simulink model "simulink_final"  (R2021a)
settings: Solver=FixedStepAuto  StartTime=0.0  StopTime=10.0  FixedStep=1e-3  RelTol=1e-3  EnableMultiTasking=on
undefined symbols (not defined in the file): a, A0, A1, b, c, D0, D1, D10, D11, D12, D13, D2, D3, D4, D5, D6, D7, D8, D9, magnitude, PTA0, PTA1, PTA2, PTB2, PTB23, PTB3, PTB9, PTC16, PTC17, PTC2, PTC3, PTC4, PTD0, PTD1, PTD2, PTD3
libraries: frdmk64flib x34, dspstat3 x2, hdlsllib x2, etargetslib x2, simulink x1
settings Model: ExtModeTrigDuration=5  Creator=14610  LastModifiedBy=微星
settings SolverCC: AlgebraicLoopSolver=TrustRegion
settings OptimizationCC: EnhancedBackFolding=on  PassReuseOutputArgsAs=Individual arguments  ZeroExternalMemoryAtStartup=off  ZeroInternalMemoryAtStartup=off  MaxStackSize=64  OptimizeBlockOrder=speed  DifferentSizesBufferReuse=on  OptimizationCustomize=off  EfficientTunableParamExpr=on
settings DebuggingCC: ParameterTunabilityLossMsg=error  SFMachineParentedDataDiag=warning
settings HardwareCC: ProdBitPerPointer=32  ProdBitPerSizeT=32  ProdBitPerPtrDiffT=32  ProdLargestAtomicInteger=Long  ProdLargestAtomicFloat=Double  ProdWordSize=32  ProdHWDeviceType=ARM Compatible->ARM Cortex  UseEmbeddedCoderFeatures=off
settings SFSimCC: MATLABDynamicMemAlloc=off
settings RTWCC: SystemTargetFile=ert.tlc  HardwareBoard=NXP FRDM-K64F  TLCOptions="-aInlineSetEventsForThisBaseRateFcn=TLC_FALSE -aSuppressMultiTaskScheduler=TLC_FALSE  -aRateBasedStepFcn=0"  TemplateMakefile=ert_default_tmf  Toolchain=GNU Tools for ARM Embedded Processors
settings CodeAppCC: ForceParamTrailComments=on  IgnoreCustomStorageClasses=off  OperatorAnnotations=on  SimulinkDataObjDesc=on  SFDataObjDesc=on  InsertBlockDesc=on
settings ERTTargetCC: SupportNonInlinedSFcns=on

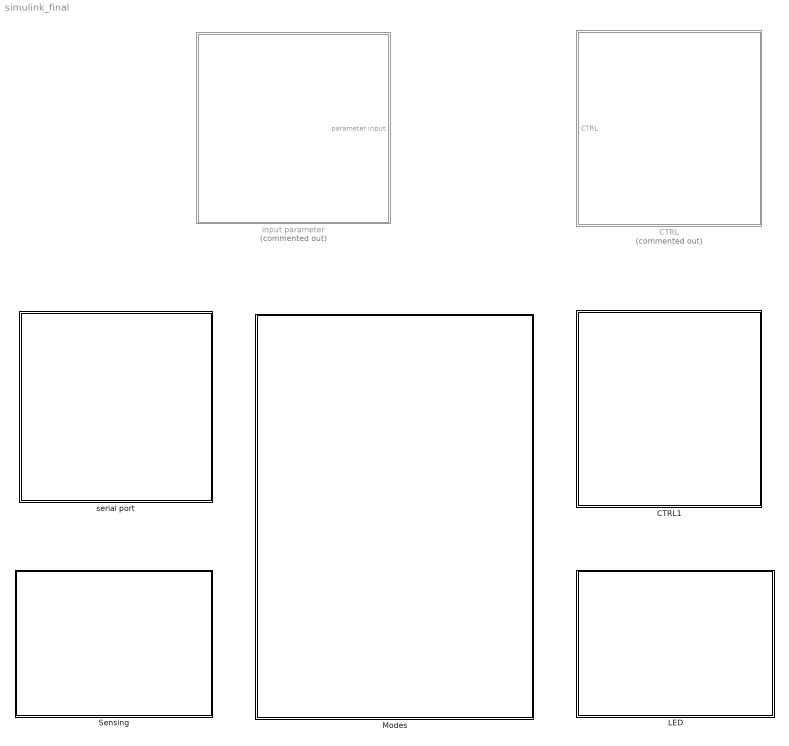
== system simulink_final ==
  CTRL : Subsystem  Commented=on
  CTRL1 : Subsystem
  LED : Subsystem
  Modes : Subsystem
  Sensing : Subsystem
  input parameter : Subsystem  Commented=on
  serial port : Subsystem

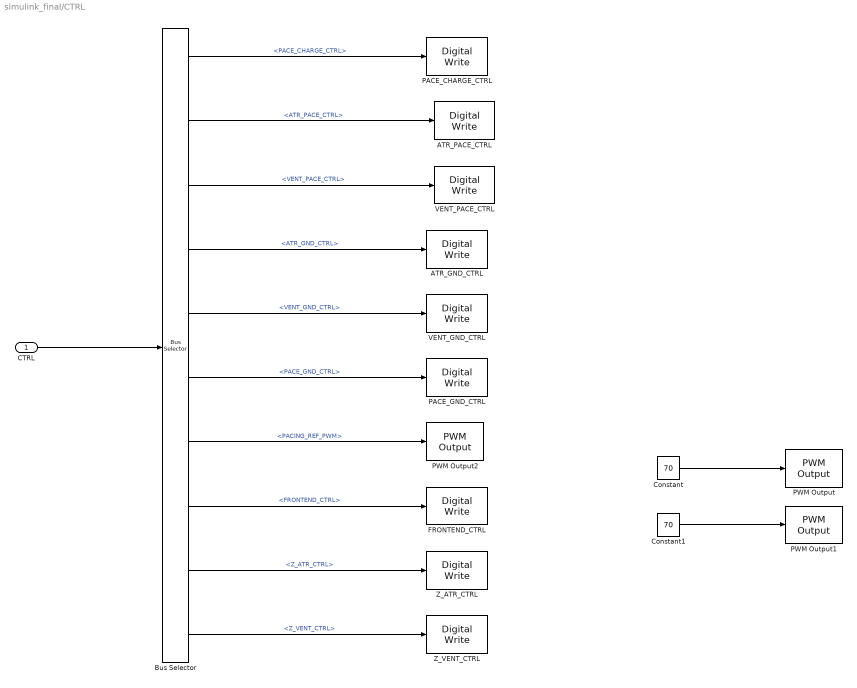
== system simulink_final/CTRL ==
  CTRL : Inport
  ATR_GND_CTRL : frdmk64flib/Digital Write  Whichpin=PTD2 (D11)
  ATR_PACE_CTRL : frdmk64flib/Digital Write  Whichpin=PTA0 (D8)
  Bus Selector : BusSelector  OutputSignals=PACE_CHARGE_CTRL,ATR_PACE_CTRL,VENT_PACE_CTRL,ATR_GND_CTRL,VENT_GND_CTRL,PACE_GND_CTRL,PACING_REF_PWM,FRONTEND_CTRL,Z_ATR_CTRL,Z_VENT_CTRL
  Constant : Constant  Value=70
  Constant1 : Constant  Value=70
  FRONTEND_CTRL : frdmk64flib/Digital Write  Whichpin=PTD1 (D13)
  PACE_CHARGE_CTRL : frdmk64flib/Digital Write  Whichpin=PTB9 (D2)
  PACE_GND_CTRL : frdmk64flib/Digital Write  Whichpin=PTD0 (D10)
  PWM Output : frdmk64flib/PWM Output  Whichpin=PTC2 (D6)  InitialFrequency=2000  InitialDutyCycle=30
  PWM Output1 : frdmk64flib/PWM Output  Whichpin=PTA1 (D3)  InitialFrequency=2000  InitialDutyCycle=30
  PWM Output2 : frdmk64flib/PWM Output  Whichpin=PTA2 (D5)  InitialFrequency=2000  InitialDutyCycle=30
  VENT_GND_CTRL : frdmk64flib/Digital Write  Whichpin=PTD3 (D12)
  VENT_PACE_CTRL : frdmk64flib/Digital Write  Whichpin=PTC4 (D9)
  Z_ATR_CTRL : frdmk64flib/Digital Write  Whichpin=PTB23 (D4)
  Z_VENT_CTRL : frdmk64flib/Digital Write  Whichpin=PTC3 (D7)
  wires:
  CTRL/1 -> Bus Selector/1
  Bus Selector/2 -> ATR_PACE_CTRL/1  "<ATR_PACE_CTRL>"
  Bus Selector/1 -> PACE_CHARGE_CTRL/1  "<PACE_CHARGE_CTRL>"
  Bus Selector/3 -> VENT_PACE_CTRL/1  "<VENT_PACE_CTRL>"
  Bus Selector/4 -> ATR_GND_CTRL/1  "<ATR_GND_CTRL>"
  Bus Selector/5 -> VENT_GND_CTRL/1  "<VENT_GND_CTRL>"
  Bus Selector/6 -> PACE_GND_CTRL/1  "<PACE_GND_CTRL>"
  Bus Selector/7 -> PWM Output2/1  "<PACING_REF_PWM>"
  Bus Selector/8 -> FRONTEND_CTRL/1  "<FRONTEND_CTRL>"
  Bus Selector/9 -> Z_ATR_CTRL/1  "<Z_ATR_CTRL>"
  Bus Selector/10 -> Z_VENT_CTRL/1  "<Z_VENT_CTRL>"
  Constant/1 -> PWM Output/1
  Constant1/1 -> PWM Output1/1

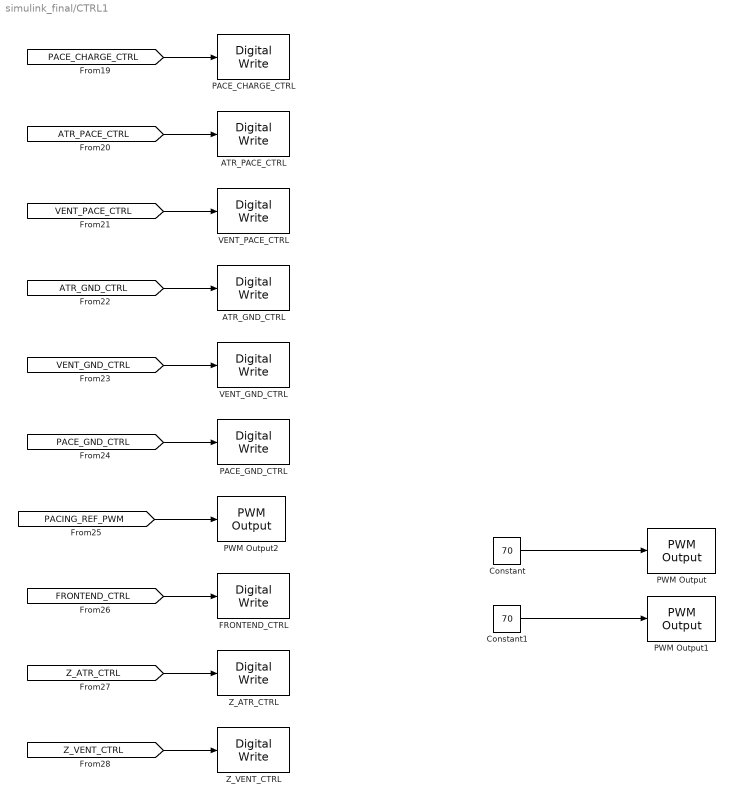
== system simulink_final/CTRL1 ==
  ATR_GND_CTRL : frdmk64flib/Digital Write  Whichpin=PTD2 (D11)
  ATR_PACE_CTRL : frdmk64flib/Digital Write  Whichpin=PTA0 (D8)
  Constant : Constant  Value=70
  Constant1 : Constant  Value=70
  FRONTEND_CTRL : frdmk64flib/Digital Write  Whichpin=PTD1 (D13)
  PACE_CHARGE_CTRL : frdmk64flib/Digital Write  Whichpin=PTB9 (D2)
  PACE_GND_CTRL : frdmk64flib/Digital Write  Whichpin=PTD0 (D10)
  PWM Output : frdmk64flib/PWM Output  Whichpin=PTC2 (D6)  InitialFrequency=2000  InitialDutyCycle=30
  PWM Output1 : frdmk64flib/PWM Output  Whichpin=PTA1 (D3)  InitialFrequency=2000  InitialDutyCycle=30
  PWM Output2 : frdmk64flib/PWM Output  Whichpin=PTA2 (D5)  InitialFrequency=2000  InitialDutyCycle=30
  VENT_GND_CTRL : frdmk64flib/Digital Write  Whichpin=PTD3 (D12)
  VENT_PACE_CTRL : frdmk64flib/Digital Write  Whichpin=PTC4 (D9)
  Z_ATR_CTRL : frdmk64flib/Digital Write  Whichpin=PTB23 (D4)
  Z_VENT_CTRL : frdmk64flib/Digital Write  Whichpin=PTC3 (D7)
  wires:
  Constant/1 -> PWM Output/1
  Constant1/1 -> PWM Output1/1
  [PACE_CHARGE_CTRL] -> PACE_CHARGE_CTRL/1
  [ATR_PACE_CTRL] -> ATR_PACE_CTRL/1
  [VENT_PACE_CTRL] -> VENT_PACE_CTRL/1
  [ATR_GND_CTRL] -> ATR_GND_CTRL/1
  [VENT_GND_CTRL] -> VENT_GND_CTRL/1
  [PACE_GND_CTRL] -> PACE_GND_CTRL/1
  [Z_VENT_CTRL] -> Z_VENT_CTRL/1
  [FRONTEND_CTRL] -> FRONTEND_CTRL/1
  [Z_ATR_CTRL] -> Z_ATR_CTRL/1
  [PACING_REF_PWM] -> PWM Output2/1

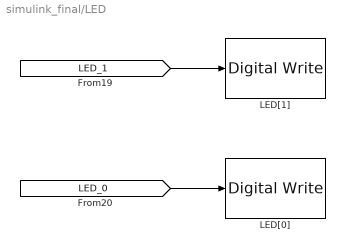
== system simulink_final/LED ==
  LED[0] : frdmk64flib/Digital Write  Whichpin=RED_LED
  LED[1] : frdmk64flib/Digital Write  Whichpin=GREEN_LED
  wires:
  [LED_1] -> LED[1]/1
  [LED_0] -> LED[0]/1

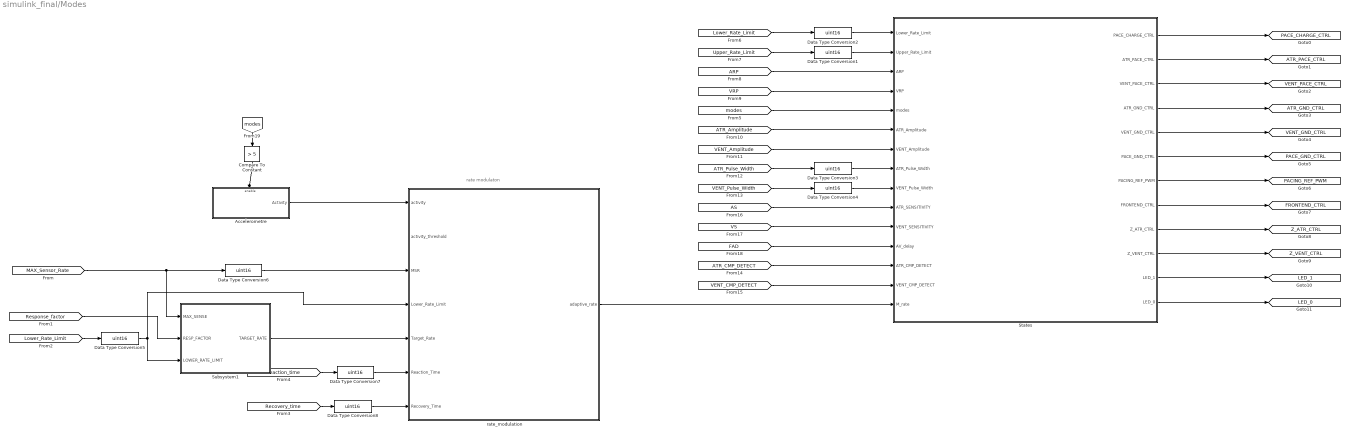
== system simulink_final/Modes ==
  note: rate modulaton
  Accelerometre : Subsystem
  Compare To Constant : simulink/Logic and Bit Operations/Compare To Constant  relop=>  const=5  OutDataTypeStr=boolean
  Data Type Conversion{1..8} (8 alike) : DataTypeConversion  OutDataTypeStr=uint16
  States : Stateflow chart
      settings: PortSchema="{\"entries\":[{\"content\":{\"sides\":[{\"content\":{\"connectorIds\":[\"In1\",\"In2\",\"In3\",\"In4\",\"In5\",\"In8\",\"In9\",\"In10\",\"In11\",\"In13\",\"In14\",\"In12\",\"In6\",\"In7\",\"In15\"]},\"type\":\"ConnectorPlacement.EquallySpacedRectSide\",\"uuid\":\"1bf89235-5b2a-4a6d-8fd1-80cb7ace4fe1\"},{\"content\":{\"connectorIds\":[\"Out1\",\"Out2\",\"Out3\",\"Out4\",\"Out5\",\"Out6\",\"Out7\",\"Out8\",\"Out9\",\"Out10\",\"Out11\",\"Out12\"],\"side\":\"RIGHT\"},\"type\":\"ConnectorPlacement.EquallySpacedRectSide\",\"uuid\":\"14ca63ff-77f8-4fed-b6c6-f39543f8346a\"},{\"content\":{\"connectorIds\":[],\"side\":\"TOP\"},\"type\":\"ConnectorPlacement.EquallySpacedRectSide\",\"uuid\":\"86655f59-e294-4cfd-9413-44776565e2db\"}]},\"type\":\"ConnectorPlacement.EquallySpacedConnector\",\"uuid\":\"c44c9a5a-010f-4149-9f0b-fe431661db61\"}],\"packageUris\":[\"http://schema.mathworks.com/mf0/Connector/R2020b\"],\"version\":\"1.0\"}"
  Subsystem1 : Subsystem
  rate_modulation : Stateflow chart  TreatAsAtomicUnit=on
  tag scope: ATR_GND_CTRL=global, ATR_PACE_CTRL=global, FRONTEND_CTRL=global, LED_0=global, LED_1=global, PACE_CHARGE_CTRL=global, PACE_GND_CTRL=global, PACING_REF_PWM=global, VENT_GND_CTRL=global, VENT_PACE_CTRL=global, Z_ATR_CTRL=global, Z_VENT_CTRL=global
  wires:
  [modes] -> States/5(modes)
  [VRP] -> States/4(VRP)
  [ARP] -> States/3(ARP)
  [VENT_Pulse_Width] -> Data Type Conversion4/1
  [VENT_Amplitude] -> States/9(VENT_Amplitude)
  [ATR_Amplitude] -> States/8(ATR_Amplitude)
  [Upper_Rate_Limit] -> Data Type Conversion1/1
  [Lower_Rate_Limit] -> Data Type Conversion2/1
  States/1(PACE_CHARGE_CTRL) -> [PACE_CHARGE_CTRL]
  States/2(ATR_PACE_CTRL) -> [ATR_PACE_CTRL]
  States/3(VENT_PACE_CTRL) -> [VENT_PACE_CTRL]
  States/4(ATR_GND_CTRL) -> [ATR_GND_CTRL]
  States/5(VENT_GND_CTRL) -> [VENT_GND_CTRL]
  States/6(PACE_GND_CTRL) -> [PACE_GND_CTRL]
  States/7(PACING_REF_PWM) -> [PACING_REF_PWM]
  States/8(FRONTEND_CTRL) -> [FRONTEND_CTRL]
  States/9(Z_ATR_CTRL) -> [Z_ATR_CTRL]
  States/10(Z_VENT_CTRL) -> [Z_VENT_CTRL]
  [ATR_Pulse_Width] -> Data Type Conversion3/1
  [AS] -> States/13(ATR_SENSITIVITY)
  [VS] -> States/14(VENT_SENSITIVITY)
  [FAD] -> States/12(AV_delay)
  [MAX_Sensor_Rate] -> Subsystem1/1(MAX_SENSE), Data Type Conversion6/1
  [Response_factor] -> Subsystem1/2(RESP_FACTOR)
  [Lower_Rate_Limit] -> Data Type Conversion5/1
  [ATR_CMP_DETECT] -> States/6(ATR_CMP_DETECT)
  [VENT_CMP_DETECT] -> States/7(VENT_CMP_DETECT)
  States/11(LED_1) -> [LED_1]
  States/12(LED_0) -> [LED_0]
  [modes] -> Compare To Constant/1
  Compare To Constant/1 -> Accelerometre/Enable
  Data Type Conversion2/1 -> States/1(Lower_Rate_Limit)
  Data Type Conversion1/1 -> States/2(Upper_Rate_Limit)
  Data Type Conversion3/1 -> States/10(ATR_Pulse_Width)
  Data Type Conversion4/1 -> States/11(VENT_Pulse_Width)
  Data Type Conversion5/1 -> Subsystem1/3(LOWER_RATE_LIMIT), rate_modulation/4(Lower_Rate_Limit)
  Accelerometre/1(Activity) -> rate_modulation/1(activity)
  Subsystem1/1(TARGET_RATE) -> rate_modulation/5(Target_Rate)
  [Reaction_time] -> Data Type Conversion7/1
  [Recovery_time] -> Data Type Conversion8/1
  Data Type Conversion6/1 -> rate_modulation/3(MSR)
  Data Type Conversion7/1 -> rate_modulation/6(Reaction_Time)
  Data Type Conversion8/1 -> rate_modulation/7(Recovery_Time)
  rate_modulation/1(adaptive_rate) -> States/15(M_rate)

== system simulink_final/Sensing ==
  ATR_CMP_ DETECT : frdmk64flib/Digital Read  Whichpin=PTC16 (D0)  SampleTime=-1
  VENT_CMP_DETECT : frdmk64flib/Digital Read  Whichpin=PTC17 (D1)  SampleTime=-1
  tag scope: ATR_CMP_DETECT=global, VENT_CMP_DETECT=global
  wires:
  ATR_CMP_ DETECT/1 -> [ATR_CMP_DETECT]  "ATR_CMP_ DETECT"
  VENT_CMP_DETECT/1 -> [VENT_CMP_DETECT]  "VENT_CMP_ DETECT"

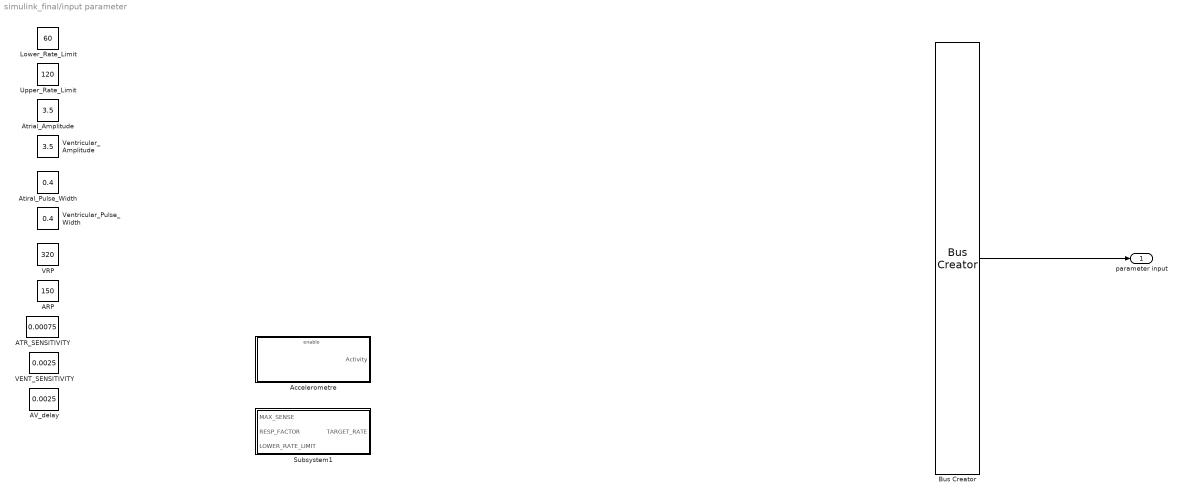
== system simulink_final/input parameter ==
  ARP : Constant  Value=150
  ATR_SENSITIVITY : Constant  Value=0.00075
  AV_delay : Constant  Value=0.0025
  Accelerometre : Subsystem
  Atiral_Pulse_Width : Constant  Value=0.4
  Atrial_Amplitude : Constant  Value=3.5
  Bus Creator : BusCreator  Inputs=12
  Lower_Rate_Limit : Constant  Value=60
  Subsystem1 : Subsystem
  Upper_Rate_Limit : Constant  Value=120
  VENT_SENSITIVITY : Constant  Value=0.0025
  VRP : Constant  Value=320
  Ventricular_Amplitude : Constant  Value=3.5
  Ventricular_Pulse_Width : Constant  Value=0.4
  parameter input : Outport
  wires:
  Bus Creator/1 -> parameter input/1
  ? -> Bus Creator/1  "modes"
  ? -> Bus Creator/2
  ? -> Bus Creator/3
  ? -> Bus Creator/4
  ? -> Bus Creator/5
  ? -> Bus Creator/6
  ? -> Bus Creator/7
  ? -> Bus Creator/8
  ? -> Bus Creator/9

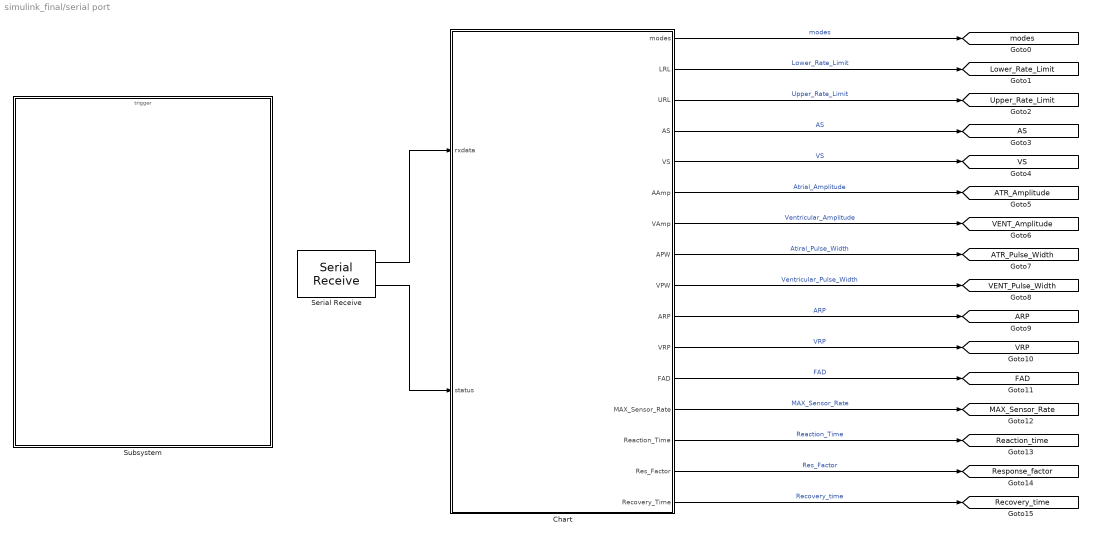
== system simulink_final/serial port ==
  Chart : Stateflow chart  TreatAsAtomicUnit=on
      settings: PortSchema="{\"entries\":[{\"content\":{\"sides\":[{\"content\":{\"connectorIds\":[\"In1\",\"In2\"]},\"type\":\"ConnectorPlacement.EquallySpacedRectSide\",\"uuid\":\"355b2c62-f4ab-4f69-b4c3-58c4813cdbb8\"},{\"content\":{\"connectorIds\":[\"Out1\",\"Out2\",\"Out14\",\"Out15\",\"Out16\",\"Out3\",\"Out4\",\"Out5\",\"Out6\",\"Out7\",\"Out8\",\"Out9\",\"Out10\",\"Out11\",\"Out12\",\"Out13\"],\"side\":\"RIGHT\"},\"type\":\"ConnectorPlacement.EquallySpacedRectSide\",\"uuid\":\"e39f9fe7-8151-4d9f-b318-f4c2a6150d39\"},{\"content\":{\"connectorIds\":[],\"side\":\"TOP\"},\"type\":\"ConnectorPlacement.EquallySpacedRectSide\",\"uuid\":\"4076b67e-1825-4591-a111-6e489612a839\"}]},\"type\":\"ConnectorPlacement.EquallySpacedConnector\",\"uuid\":\"92306b88-4ce7-4751-b58c-bc5096b575c6\"}],\"packageUris\":[\"http://schema.mathworks.com/mf0/Connector/R2020b\"],\"version\":\"1.0\"}"
  Serial Receive : frdmk64flib/Serial Receive  SCIModule=0  Baudrate=uint32(9600)  Parity=None  StopBits=1  HardwareFlowControl=None  ByteOrder=LittleEndian  DataType=uint8  DataLength=21  BlockingMode=off  OutputStatus=on  SampleTime=-1
  Subsystem : Subsystem
  tag scope: ARP=global, AS=global, ATR_Amplitude=global, ATR_Pulse_Width=global, FAD=global, Lower_Rate_Limit=global, MAX_Sensor_Rate=global, Reaction_time=global, Recovery_time=global, Response_factor=global, Upper_Rate_Limit=global, VENT_Amplitude=global, VENT_Pulse_Width=global, VRP=global, VS=global, modes=global
  wires:
  Chart/1(modes) -> [modes]  "modes"
  Chart/2(LRL) -> [Lower_Rate_Limit]  "Lower_Rate_Limit"
  Chart/14(URL) -> [Upper_Rate_Limit]  "Upper_Rate_Limit"
  Chart/15(AS) -> [AS]  "AS"
  Chart/16(VS) -> [VS]  "VS"
  Chart/3(AAmp) -> [ATR_Amplitude]  "Atrial_Amplitude"
  Chart/4(VAmp) -> [VENT_Amplitude]  "Ventricular_Amplitude"
  Chart/5(APW) -> [ATR_Pulse_Width]  "Atiral_Pulse_Width"
  Chart/6(VPW) -> [VENT_Pulse_Width]  "Ventricular_Pulse_Width"
  Chart/7(ARP) -> [ARP]  "ARP"
  Chart/8(VRP) -> [VRP]  "VRP"
  Chart/9(FAD) -> [FAD]  "FAD"
  Chart/10(MAX_Sensor_Rate) -> [MAX_Sensor_Rate]  "MAX_Sensor_Rate"
  Chart/11(Reaction_Time) -> [Reaction_time]  "Reaction_Time"
  Chart/12(Res_Factor) -> [Response_factor]  "Res_Factor"
  Chart/13(Recovery_Time) -> [Recovery_time]  "Recovery_time"
  Serial Receive/1 -> Chart/1(rxdata)
  Serial Receive/2 -> Chart/2(status)

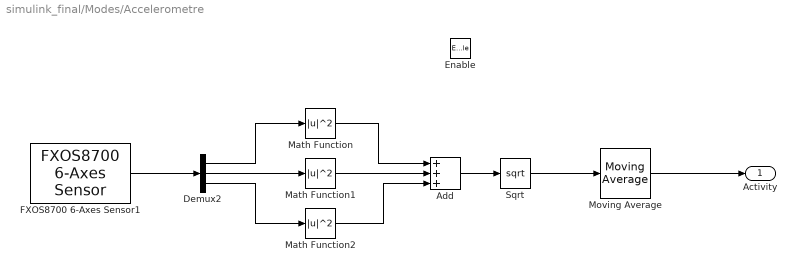
== system simulink_final/Modes/Accelerometre ==
  Enable : EnablePort
  Add : Sum  Inputs=+++
  Demux2 : Demux  Outputs=3
  FXOS8700 6-Axes Sensor1 : frdmk64flib/FXOS8700 6-Axes Sensor  Activesensor=Accelerometer only  ODR=100Hz  HybridODR=400Hz  Accelfullrange=-4g to +4g  SampleTime=1/100
  Math Function : Math  Operator=magnitude^2  SignedPower=on  OutDataTypeStr=double  SaturateOnIntegerOverflow=on
  Math Function1 : Math  Operator=magnitude^2  SignedPower=on  OutDataTypeStr=double  SaturateOnIntegerOverflow=on
  Math Function2 : Math  Operator=magnitude^2  SignedPower=on  OutDataTypeStr=double  SaturateOnIntegerOverflow=on
  Moving Average : dspstat3/Moving Average  Method=Sliding window  ForgettingFactorPort=off  SpecifyWindowLength=on  WindowLength=4  ForgettingFactor=0.9  SimulateUsing=Code generation
  Sqrt : Sqrt  SaturateOnIntegerOverflow=on
  Activity : Outport  OutDataTypeStr=double  SourceOfInitialOutputValue=Input signal
  wires:
  Sqrt/1 -> Moving Average/1
  FXOS8700 6-Axes Sensor1/1 -> Demux2/1
  Math Function/1 -> Add/1
  Add/1 -> Sqrt/1
  Math Function2/1 -> Add/3
  Demux2/2 -> Math Function1/1
  Math Function1/1 -> Add/2
  Demux2/1 -> Math Function/1
  Demux2/3 -> Math Function2/1
  Moving Average/1 -> Activity/1

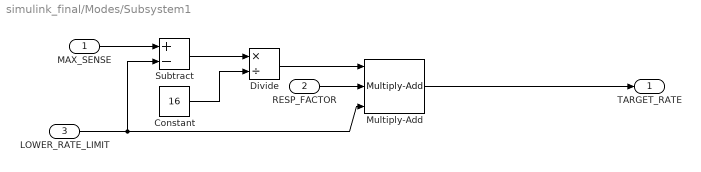
== system simulink_final/Modes/Subsystem1 ==
  MAX_SENSE : Inport
  RESP_FACTOR : Inport  Port=2
  LOWER_RATE_LIMIT : Inport  Port=3
  Constant : Constant  Value=16
  Divide : Product  Inputs=*/
  Multiply-Add : hdlsllib/HDL Operations/Multiply-Add  Function=c+(a.*b)  datatype=uint16  RndMeth=Nearest  DoSatur=off  FMA=off
      settings: SourceProductBaseCode=SL
  Subtract : Sum  Inputs=+-
  TARGET_RATE : Outport  OutDataTypeStr=uint16  SourceOfInitialOutputValue=Input signal
  wires:
  MAX_SENSE/1 -> Subtract/1
  Subtract/1 -> Divide/1
  Constant/1 -> Divide/2
  Divide/1 -> Multiply-Add/1
  RESP_FACTOR/1 -> Multiply-Add/2
  Multiply-Add/1 -> TARGET_RATE/1
  LOWER_RATE_LIMIT/1 -> Subtract/2, Multiply-Add/3

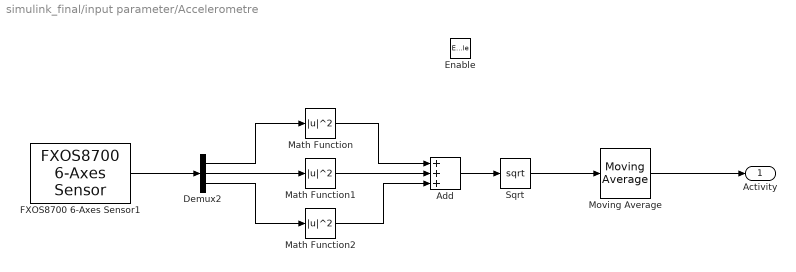
== system simulink_final/input parameter/Accelerometre ==
  Enable : EnablePort
  Add : Sum  Inputs=+++
  Demux2 : Demux  Outputs=3
  FXOS8700 6-Axes Sensor1 : frdmk64flib/FXOS8700 6-Axes Sensor  Activesensor=Accelerometer only  ODR=100Hz  HybridODR=400Hz  Accelfullrange=-4g to +4g  SampleTime=1/100
  Math Function : Math  Operator=magnitude^2  SignedPower=on  OutDataTypeStr=double  SaturateOnIntegerOverflow=on
  Math Function1 : Math  Operator=magnitude^2  SignedPower=on  OutDataTypeStr=double  SaturateOnIntegerOverflow=on
  Math Function2 : Math  Operator=magnitude^2  SignedPower=on  OutDataTypeStr=double  SaturateOnIntegerOverflow=on
  Moving Average : dspstat3/Moving Average  Method=Sliding window  ForgettingFactorPort=off  SpecifyWindowLength=on  WindowLength=4  ForgettingFactor=0.9  SimulateUsing=Code generation
  Sqrt : Sqrt  SaturateOnIntegerOverflow=on
  Activity : Outport  OutDataTypeStr=double  SourceOfInitialOutputValue=Input signal
  wires:
  Sqrt/1 -> Moving Average/1
  FXOS8700 6-Axes Sensor1/1 -> Demux2/1
  Math Function/1 -> Add/1
  Add/1 -> Sqrt/1
  Math Function2/1 -> Add/3
  Demux2/2 -> Math Function1/1
  Math Function1/1 -> Add/2
  Demux2/1 -> Math Function/1
  Demux2/3 -> Math Function2/1
  Moving Average/1 -> Activity/1

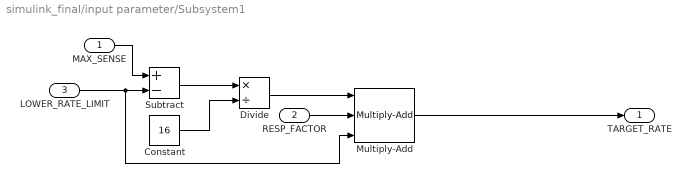
== system simulink_final/input parameter/Subsystem1 ==
  MAX_SENSE : Inport
  RESP_FACTOR : Inport  Port=2
  LOWER_RATE_LIMIT : Inport  Port=3
  Constant : Constant  Value=16
  Divide : Product  Inputs=*/
  Multiply-Add : hdlsllib/HDL Operations/Multiply-Add  Function=c+(a.*b)  datatype=uint16  RndMeth=Nearest  DoSatur=off  FMA=off
      settings: SourceProductBaseCode=SL
  Subtract : Sum  Inputs=+-
  TARGET_RATE : Outport  OutDataTypeStr=uint16  SourceOfInitialOutputValue=Input signal
  wires:
  MAX_SENSE/1 -> Subtract/1
  LOWER_RATE_LIMIT/1 -> Multiply-Add/3, Subtract/2
  Subtract/1 -> Divide/1
  Constant/1 -> Divide/2
  Divide/1 -> Multiply-Add/1
  RESP_FACTOR/1 -> Multiply-Add/2
  Multiply-Add/1 -> TARGET_RATE/1

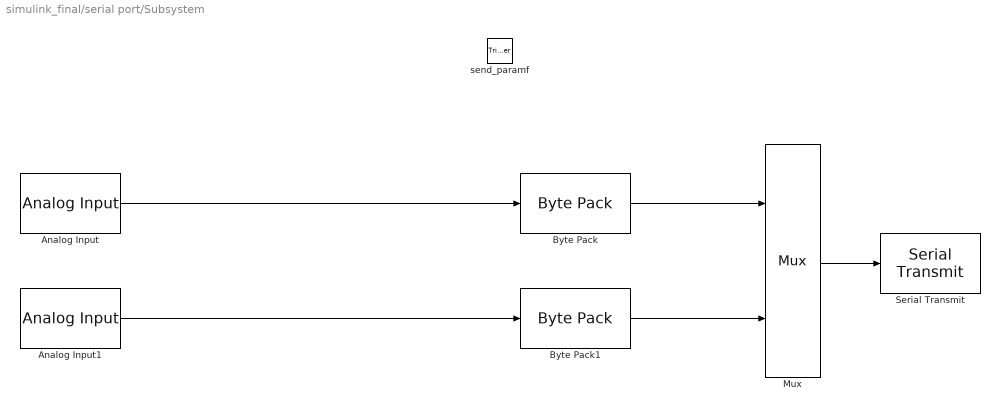
== system simulink_final/serial port/Subsystem ==
  send_paramf : TriggerPort  TriggerType=function-call  IsSimulinkFunction=on  FunctionName=send_paramf  VariantControl=(inherit)  PortDimensions=1
  Analog Input : frdmk64flib/Analog Input  Whichpin=PTB2 (A0)  SampleTime=-1
  Analog Input1 : frdmk64flib/Analog Input  Whichpin=PTB3 (A1)  SampleTime=-1
  Byte Pack : etargetslib/Byte Pack  datatypes={'double'}  byteAlign=1
  Byte Pack1 : etargetslib/Byte Pack  datatypes={'double'}  byteAlign=1
  Mux : Mux  Inputs=2
  Serial Transmit : frdmk64flib/Serial Transmit  SCIModule=0  Baudrate=uint32(9600)  Parity=None  StopBits=1  HardwareFlowControl=None  ByteOrder=LittleEndian  BlockingMode=on  OutputStatus=off
  wires:
  Byte Pack/1 -> Mux/1
  Byte Pack1/1 -> Mux/2
  Mux/1 -> Serial Transmit/1
  Analog Input/1 -> Byte Pack/1
  Analog Input1/1 -> Byte Pack1/1

== stateflow chart simulink_final/Modes/States ==
  note: will leave the defult state if recieve any changes in parameter mode
  state Defult
    entry:
    PACE_CHARGE_CTRL=0;
    PACE_GND_CTRL = 0;
    ATR_PACE_CTRL = 0;
    ATR_GND_CTRL = 0;
    VENT_PACE_CTRL = 0;
    VENT_GND_CTRL = 0;
    LED_1 = 1;
    %ATR_CMP_REF_PWM = ATR_SENSITIVITY*100/3.3;
    %VENT_CMP_REF_PWM = VENT_SENSITIVITY*100/3.3;
  note: will go back to defult sate if the any new changes in parameter mode
  state AAIR
    state AAIR
      entry:
      PACE_CHARGE_CTRL=1;
      PACE_GND_CTRL = 1;
      ATR_PACE_CTRL = 0;
      ATR_GND_CTRL = 1;
      VENT_PACE_CTRL = 0;
      VENT_GND_CTRL = 0;
      PACING_REF_PWM = ATR_Amplitude;
      FRONTEND_CTRL = 1;
      Z_ATR_CTRL = 0;
      Z_VENT_CTRL = 0;
      LED_0 = 0;
      LED_1 = 0;
    note: charging C22 for the atrium pacing
    state Refractory_ATR
      entry:
      PACE_CHARGE_CTRL=1;
      PACE_GND_CTRL = 1;
      ATR_PACE_CTRL = 0;
      ATR_GND_CTRL = 1;
      VENT_PACE_CTRL = 0;
      VENT_GND_CTRL = 0;
      PACING_REF_PWM = ATR_Amplitude;
      FRONTEND_CTRL = 1;
      Z_ATR_CTRL = 0;
      Z_VENT_CTRL = 0;
      LED_0 = 0;
    state AAIR_PACING
      entry:
      PACE_CHARGE_CTRL=0;
      PACE_GND_CTRL = 1;
      ATR_PACE_CTRL = 1;
      ATR_GND_CTRL = 0;
      Z_ATR_CTRL = 0;
      Z_VENT_CTRL = 0;
      VENT_PACE_CTRL = 0;
      VENT_GND_CTRL = 0;
      LED_0 = 1;
    AAIR_PACING -> AAIR.AAIR : after(ATR_Pulse_Width,msec)
    AAIR.Refractory_ATR -> AAIR.AAIR [order 2] : [ATR_CMP_DETECT==1]
    AAIR.AAIR -> AAIR.Refractory_ATR [order 1] : after(ARP,msec)
    AAIR.Refractory_ATR -> AAIR_PACING [order 1] : after(60/M_rate * 1000 - ARP - ATR_Pulse_Width,msec)
  state VVIR
    state VVIR
      entry:
      PACE_CHARGE_CTRL=1;
      PACE_GND_CTRL = 1;
      ATR_PACE_CTRL = 0;
      ATR_GND_CTRL = 0;
      VENT_PACE_CTRL = 0;
      VENT_GND_CTRL = 1;
      PACING_REF_PWM = VENT_Amplitude;
      FRONTEND_CTRL = 1;
      Z_ATR_CTRL = 0;
      Z_VENT_CTRL = 0;
      LED_0 = 0;
      LED_1 = 0;
    note: charging C22 for the ventricle pacing
    state Refractory_VENT
      entry:
      PACE_CHARGE_CTRL=1;
      PACE_GND_CTRL = 1;
      ATR_PACE_CTRL = 0;
      ATR_GND_CTRL = 0;
      VENT_PACE_CTRL = 0;
      VENT_GND_CTRL = 1;
      PACING_REF_PWM = VENT_Amplitude;
      FRONTEND_CTRL = 1;
      Z_ATR_CTRL = 0;
      Z_VENT_CTRL = 0;
      LED_0 = 0;
    state VVIR_PACING
      entry:
      PACE_CHARGE_CTRL=0;
      PACE_GND_CTRL = 1;
      ATR_PACE_CTRL = 0;
      ATR_GND_CTRL = 0;
      Z_ATR_CTRL = 0;
      Z_VENT_CTRL = 0;
      VENT_PACE_CTRL = 1;
      VENT_GND_CTRL = 0;
      LED_0 = 1;
    VVIR.Refractory_VENT -> VVIR.VVIR [order 1] : [VENT_CMP_DETECT==1]
    VVIR_PACING -> VVIR.VVIR : after(VENT_Pulse_Width,msec)
    VVIR.VVIR -> VVIR.Refractory_VENT [order 2] : after(VRP,msec)
    VVIR.Refractory_VENT -> VVIR_PACING [order 2] : after(60/M_rate * 1000 - VRP - VENT_Pulse_Width,msec)
  state AOO
    state AOO
      entry:
      ATR_PACE_CTRL = 0;
      VENT_PACE_CTRL = 0;
      PACING_REF_PWM = ATR_Amplitude;
      PACE_CHARGE_CTRL = 1;
      PACE_GND_CTRL = 1;
      Z_ATR_CTRL = 0;
      Z_VENT_CTRL = 0;
      ATR_GND_CTRL = 1;
      VENT_GND_CTRL = 0;
      FRONTEND_CTRL = 0;
      LED_0 = 0;
      LED_1 = 0;
    note: charging C22 for the atrium pacing
    state AOO_PACING
      entry:
      PACE_CHARGE_CTRL=0;
      PACE_GND_CTRL = 1;
      ATR_PACE_CTRL = 1;
      ATR_GND_CTRL = 0;
      Z_ATR_CTRL = 0;
      Z_VENT_CTRL = 0;
      VENT_PACE_CTRL = 0;
      VENT_GND_CTRL = 0;
      LED_0 = 1;
    AOO.AOO -> AOO_PACING [order 2] : after(60000/Lower_Rate_Limit-ATR_Pulse_Width,msec)
    AOO_PACING -> AOO.AOO : after(ATR_Pulse_Width,msec)
  state VOO
    state VOO
      entry:
      ATR_PACE_CTRL = 0;
      VENT_PACE_CTRL = 0;
      PACING_REF_PWM = VENT_Amplitude;
      PACE_CHARGE_CTRL = 1;
      PACE_GND_CTRL = 1;
      Z_ATR_CTRL = 0;
      Z_VENT_CTRL = 0;
      ATR_GND_CTRL = 0;
      VENT_GND_CTRL = 1;
      FRONTEND_CTRL = 0;
      LED_0 = 0;
      LED_1 = 0;
    note: charging C22 for the ventricle pacing
    state VOO_PACING
      entry:
      PACE_CHARGE_CTRL=0;
      PACE_GND_CTRL = 1;
      ATR_PACE_CTRL = 0;
      ATR_GND_CTRL = 0;
      Z_ATR_CTRL = 0;
      Z_VENT_CTRL = 0;
      VENT_PACE_CTRL = 1;
      VENT_GND_CTRL = 0;
      LED_0 = 1;
    VOO.VOO -> VOO_PACING [order 2] : after(60000/Lower_Rate_Limit-VENT_Pulse_Width,msec)
    VOO_PACING -> VOO.VOO : after(VENT_Pulse_Width,msec)
  state AAI
    state AAI
      entry:
      PACE_CHARGE_CTRL=1;
      PACE_GND_CTRL = 1;
      ATR_PACE_CTRL = 0;
      ATR_GND_CTRL = 1;
      VENT_PACE_CTRL = 0;
      VENT_GND_CTRL = 0;
      PACING_REF_PWM = ATR_Amplitude;
      FRONTEND_CTRL = 1;
      Z_ATR_CTRL = 0;
      Z_VENT_CTRL = 0;
      LED_0 = 0;
      LED_1 = 0;
    note: charging C22 for the atrium pacing
    state Refractory_ATR
      entry:
      PACE_CHARGE_CTRL=1;
      PACE_GND_CTRL = 1;
      ATR_PACE_CTRL = 0;
      ATR_GND_CTRL = 1;
      VENT_PACE_CTRL = 0;
      VENT_GND_CTRL = 0;
      PACING_REF_PWM = ATR_Amplitude;
      FRONTEND_CTRL = 1;
      Z_ATR_CTRL = 0;
      Z_VENT_CTRL = 0;
      LED_0 = 0;
    state AAI_PACING
      entry:
      PACE_CHARGE_CTRL=0;
      PACE_GND_CTRL = 1;
      ATR_PACE_CTRL = 1;
      ATR_GND_CTRL = 0;
      Z_ATR_CTRL = 0;
      Z_VENT_CTRL = 0;
      VENT_PACE_CTRL = 0;
      VENT_GND_CTRL = 0;
      LED_0 = 1;
    AAI_PACING -> AAI.AAI : after(ATR_Pulse_Width,msec)
    AAI.Refractory_ATR -> AAI.AAI [order 2] : [ATR_CMP_DETECT==1]
    AAI.AAI -> AAI.Refractory_ATR [order 1] : after(ARP,msec)
    AAI.Refractory_ATR -> AAI_PACING [order 1] : after(60/Lower_Rate_Limit * 1000 - ARP - ATR_Pulse_Width,msec)
  state VVI
    state VVI
      entry:
      PACE_CHARGE_CTRL=1;
      PACE_GND_CTRL = 1;
      ATR_PACE_CTRL = 0;
      ATR_GND_CTRL = 0;
      VENT_PACE_CTRL = 0;
      VENT_GND_CTRL = 1;
      PACING_REF_PWM = VENT_Amplitude;
      FRONTEND_CTRL = 1;
      Z_ATR_CTRL = 0;
      Z_VENT_CTRL = 0;
      LED_0 = 0;
      LED_1 = 0;
    note: charging C22 for the ventricle pacing
    state Refractory_VENT
      entry:
      PACE_CHARGE_CTRL=1;
      PACE_GND_CTRL = 1;
      ATR_PACE_CTRL = 0;
      ATR_GND_CTRL = 0;
      VENT_PACE_CTRL = 0;
      VENT_GND_CTRL = 1;
      PACING_REF_PWM = VENT_Amplitude;
      FRONTEND_CTRL = 1;
      Z_ATR_CTRL = 0;
      Z_VENT_CTRL = 0;
      LED_0 = 0;
    state VVI_PACING
      entry:
      PACE_CHARGE_CTRL=0;
      PACE_GND_CTRL = 1;
      ATR_PACE_CTRL = 0;
      ATR_GND_CTRL = 0;
      Z_ATR_CTRL = 0;
      Z_VENT_CTRL = 0;
      VENT_PACE_CTRL = 1;
      VENT_GND_CTRL = 0;
      LED_0 = 1;
    VVI.Refractory_VENT -> VVI.VVI [order 1] : [VENT_CMP_DETECT==1]
    VVI_PACING -> VVI.VVI : after(VENT_Pulse_Width,msec)
    VVI.VVI -> VVI.Refractory_VENT [order 2] : after(VRP,msec)
    VVI.Refractory_VENT -> VVI_PACING [order 2] : after(60/Lower_Rate_Limit * 1000 - VRP - VENT_Pulse_Width,msec)
  state DOO
    note: charging C22 for the atrium pacing
    state ATR_CHARGING
      during:
      %Begin Charging C22 Capacitor
      ATR_PACE_CTRL = 0
      VENT_PACE_CTRL = 0
      PACING_REF_PWM = ATR_Amplitude
      PACE_CHARGE_CTRL = 1
      %Begin Discharging C21 Blocking Capacitor
      PACE_GND_CTRL = 1
      VENT_PACE_CTRL = 0
      Z_ATR_CTRL = 0
      Z_VENT_CTRL = 0
      ATR_PACE_CTRL = 0
      ATR_GND_CTRL = 1
      VENT_GND_CTRL = 0
    state VENT_CHARGING
      during:
      %Begin Charging C22 Capacitor
      ATR_PACE_CTRL = 0
      VENT_PACE_CTRL = 0
      PACING_REF_PWM = VENT_Amplitude
      PACE_CHARGE_CTRL = 1
      %Begin Discharging C21 Blocking Capacitor
      PACE_GND_CTRL = 1
      VENT_PACE_CTRL = 0
      Z_ATR_CTRL = 0
      Z_VENT_CTRL = 0
      ATR_PACE_CTRL = 0
      ATR_GND_CTRL = 0
      VENT_GND_CTRL = 1
    state ATR_DISCHARGING
      during:
      %Discharge C22 into Atrium (AtrialPacing)
      %Begin Charging C21 Blocking Capacitor
      PACE_CHARGE_CTRL = 0
      PACE_GND_CTRL = 1
      ATR_PACE_CTRL = 1
      ATR_GND_CTRL = 0
      Z_ATR_CTRL = 0
      Z_VENT_CTRL = 0
      VENT_GND_CTRL = 0
      VENT_PACE_CTRL  = 0
    state VENT_DISCHARGING
      during:
      %Discharge C22 into Ventricle (Vent Pacing)
      %Begin Charging Blocking Capacitor
      PACE_CHARGE_CTRL = 0
      PACE_GND_CTRL = 1
      ATR_PACE_CTRL = 0
      ATR_GND_CTRL = 0
      Z_ATR_CTRL = 0
      Z_VENT_CTRL = 0
      VENT_GND_CTRL = 0
      VENT_PACE_CTRL  = 1
    note: charging C22 for the ventricle pacing
    DOO.VENT_DISCHARGING -> DOO.VENT_CHARGING : after(VENT_Pulse_Width,msec)
    DOO.ATR_DISCHARGING -> DOO.ATR_CHARGING : after(ATR_Pulse_Width, msec)
    DOO.ATR_CHARGING -> DOO.VENT_DISCHARGING : after(AV_delay -ATR_Pulse_Width,msec)
    DOO.VENT_CHARGING -> DOO.ATR_DISCHARGING [order 1] : after(60000/Lower_Rate_Limit - VENT_Pulse_Width - AV_delay, msec)
  state AOOR
    state AOOR
      entry:
      ATR_PACE_CTRL = 0;
      VENT_PACE_CTRL = 0;
      PACING_REF_PWM = ATR_Amplitude;
      PACE_CHARGE_CTRL = 1;
      PACE_GND_CTRL = 1;
      Z_ATR_CTRL = 0;
      Z_VENT_CTRL = 0;
      ATR_GND_CTRL = 1;
      VENT_GND_CTRL = 0;
      FRONTEND_CTRL = 0;
      LED_0 = 0;
      LED_1 = 0;
    note: charging C22 for the atrium pacing
    state AOOR_PACING
      entry:
      PACE_CHARGE_CTRL=0;
      PACE_GND_CTRL = 1;
      ATR_PACE_CTRL = 1;
      ATR_GND_CTRL = 0;
      Z_ATR_CTRL = 0;
      Z_VENT_CTRL = 0;
      VENT_PACE_CTRL = 0;
      VENT_GND_CTRL = 0;
      LED_0 = 1;
    AOOR.AOOR -> AOOR_PACING [order 1] : after(60000/M_rate-ATR_Pulse_Width,msec)
    AOOR_PACING -> AOOR.AOOR : after(ATR_Pulse_Width,msec)
  state VOOR
    state VOOR
      entry:
      ATR_PACE_CTRL = 0;
      VENT_PACE_CTRL = 0;
      PACING_REF_PWM = VENT_Amplitude;
      PACE_CHARGE_CTRL = 1;
      PACE_GND_CTRL = 1;
      Z_ATR_CTRL = 0;
      Z_VENT_CTRL = 0;
      ATR_GND_CTRL = 0;
      VENT_GND_CTRL = 1;
      FRONTEND_CTRL = 0;
      LED_0 = 0;
      LED_1 = 0;
    note: charging C22 for the ventricle pacing
    state VOOR_PACING
      entry:
      PACE_CHARGE_CTRL=0;
      PACE_GND_CTRL = 1;
      ATR_PACE_CTRL = 0;
      ATR_GND_CTRL = 0;
      Z_ATR_CTRL = 0;
      Z_VENT_CTRL = 0;
      VENT_PACE_CTRL = 1;
      VENT_GND_CTRL = 0;
      LED_0 = 1;
    VOOR.VOOR -> VOOR_PACING [order 2] : after(60000/M_rate-VENT_Pulse_Width,msec)
    VOOR_PACING -> VOOR.VOOR : after(VENT_Pulse_Width,msec)
  state DOOR
    note: charging C22 for the atrium pacing
    state ATR_CHARGING
      during:
      %Begin Charging C22 Capacitor
      ATR_PACE_CTRL = 0
      VENT_PACE_CTRL = 0
      PACING_REF_PWM = ATR_Amplitude
      PACE_CHARGE_CTRL = 1
      %Begin Discharging C21 Blocking Capacitor
      PACE_GND_CTRL = 1
      VENT_PACE_CTRL = 0
      Z_ATR_CTRL = 0
      Z_VENT_CTRL = 0
      ATR_PACE_CTRL = 0
      ATR_GND_CTRL = 1
      VENT_GND_CTRL = 0
    state VENT_CHARGING
      during:
      %Begin Charging C22 Capacitor
      ATR_PACE_CTRL = 0
      VENT_PACE_CTRL = 0
      PACING_REF_PWM = VENT_Amplitude
      PACE_CHARGE_CTRL = 1
      %Begin Discharging C21 Blocking Capacitor
      PACE_GND_CTRL = 1
      VENT_PACE_CTRL = 0
      Z_ATR_CTRL = 0
      Z_VENT_CTRL = 0
      ATR_PACE_CTRL = 0
      ATR_GND_CTRL = 0
      VENT_GND_CTRL = 1
    state ATR_DISCHARGING
      during:
      %Discharge C22 into Atrium (AtrialPacing)
      %Begin Charging C21 Blocking Capacitor
      PACE_CHARGE_CTRL = 0
      PACE_GND_CTRL = 1
      ATR_PACE_CTRL = 1
      ATR_GND_CTRL = 0
      Z_ATR_CTRL = 0
      Z_VENT_CTRL = 0
      VENT_GND_CTRL = 0
      VENT_PACE_CTRL  = 0
    state VENT_DISCHARGING
      during:
      %Discharge C22 into Ventricle (Vent Pacing)
      %Begin Charging Blocking Capacitor
      PACE_CHARGE_CTRL = 0
      PACE_GND_CTRL = 1
      ATR_PACE_CTRL = 0
      ATR_GND_CTRL = 0
      Z_ATR_CTRL = 0
      Z_VENT_CTRL = 0
      VENT_GND_CTRL = 0
      VENT_PACE_CTRL  = 1
    note: charging C22 for the ventricle pacing
    DOOR.VENT_DISCHARGING -> DOOR.VENT_CHARGING : after(VENT_Pulse_Width,msec)
    DOOR.ATR_DISCHARGING -> DOOR.ATR_CHARGING : after(ATR_Pulse_Width, msec)
    DOOR.ATR_CHARGING -> DOOR.VENT_DISCHARGING : after(AV_delay -ATR_Pulse_Width,msec)
    DOOR.VENT_CHARGING -> DOOR.ATR_DISCHARGING [order 1] : after(60000/M_rate - VENT_Pulse_Width - AV_delay, msec)
  DOOR.VENT_CHARGING -> Defult [order 2] : [modes~=6]
  Defult -> DOOR.VENT_CHARGING [order 10] : [modes == 6]
  Defult -> VVIR.VVIR [order 9] : [modes == 8]
  Defult -> VOOR.VOOR [order 3] : [modes == 10]
  Defult -> AAIR.AAIR [order 8] : [modes == 7]
  AOOR.AOOR -> Defult [order 2] : [modes ~= 9]
  Defult -> AOOR.AOOR [order 7] : [modes == 9]
  VVIR.VVIR -> Defult [order 1] : [modes ~= 8]
  VVI.VVI -> Defult [order 1] : [modes ~= 4]
  AAI.AAI -> Defult [order 2] : [modes ~=3]
  AAIR.AAIR -> Defult [order 2] : [modes ~=7]
  AOO.AOO -> Defult [order 1] : [modes ~= 1]
  VOOR.VOOR -> Defult [order 1] : [modes ~= 10]
  VOO.VOO -> Defult [order 1] : [modes ~= 2]
  (default) -> Defult
  DOO.VENT_CHARGING -> Defult [order 2] : [modes ~= 5]
  Defult -> AOO.AOO [order 2] : [modes == 1]
  Defult -> VVI.VVI [order 6] : [modes == 4]
  Defult -> DOO.VENT_CHARGING [order 1] : [modes==5]
  Defult -> VOO.VOO [order 5] : [modes == 2]
  Defult -> AAI.AAI [order 4] : [modes == 3]
  data: Lower_Rate_Limit input; Upper_Rate_Limit input; ARP input; VRP input; PACE_CHARGE_CTRL output; ATR_PACE_CTRL output; VENT_PACE_CTRL output; ATR_GND_CTRL output; VENT_GND_CTRL output; PACE_GND_CTRL output; PACING_REF_PWM output; FRONTEND_CTRL output; Z_ATR_CTRL output; Z_VENT_CTRL output; modes input; ATR_CMP_DETECT input; VENT_CMP_DETECT input; ATR_Amplitude input; VENT_Amplitude input; ATR_Pulse_Width input; VENT_Pulse_Width input; AV_delay input; LED_1 output; LED_0 output; ATR_SENSITIVITY input; VENT_SENSITIVITY input; M_rate input uint16

== stateflow chart simulink_final/Modes/rate_modulation ==
  state Default
    entry:
    current_Rate = 0;
  note: will only leave this state when activity is greate than the activity threshold
  note: the rate will need to chang if the target rate is greater than the current rate
  note: the decreament action will be done with certain amount of time determined by the recovery time
  note: the increament action will be done with certain amount of time determined by the reaction time
  state increase
    entry:
    if Target_Rate <= MSR
    adaptive_rate = Target_Rate;
    else
    adaptive_rate = MSR;
    end
  state decrease
    entry:
    if Target_Rate >= Lower_Rate_Limit
    adaptive_rate = Target_Rate;
    else
    adaptive_rate = Lower_Rate_Limit;
    end
  state S0
    entry:
    current_Rate = adaptive_rate;
  Default -> Default [order 2] : [activity < activity_threshold]
  (default) -> Default
  Default -> increase [order 1] : after(1000*(MSR-Lower_Rate_Limit)/Reaction_Time * Target_Rate,msec)[activity >= activity_threshold & Target_Rate > current_Rate]
  S0 -> Default
  Default -> decrease [order 3] : after(1000*(MSR-Lower_Rate_Limit)/Recovery_Time * Target_Rate,msec)[activity >= activity_threshold & Target_Rate < current_Rate]
  increase -> S0
  decrease -> S0
  data: activity input; activity_threshold input; MSR input; Lower_Rate_Limit input; Target_Rate input; Reaction_Time input; Recovery_Time input; current_Rate local uint16; adaptive_rate output uint16

== stateflow chart simulink_final/serial port/Chart ==
  state set1
    entry:
    modes = rxdata(3);
    LRL = rxdata(4);
    URL = rxdata(5);
    if(modes == 1)
    AAmp = rxdata(6);
    APW = typecast(rxdata(7:10),'single');
    elseif(modes == 2)
    VAmp = rxdata(6);
    VPW = typecast(rxdata(7:10),'single');
    elseif(modes == 3)
    AAmp = rxdata(6);
    APW = typecast(rxdata(7:10),'single');
    ARP = typecast(rxdata(11:12),'uint16');
    AS = typecast(rxdata(13:16),'single');
    elseif(modes == 4)
    VAmp = rxdata(6);
    VPW = typecast(rxdata(7:10),'single');
    VRP = typecast(rxdata(11:12),'uint16');
    VS = typecast(rxdata(13:16),'single');
    elseif(modes == 5)
    VAmp = rxdata(6);
    VPW = typecast(rxdata(7:10),'single');
    AAmp = rxdata(11);
    APW = typecast(rxdata(12:15),'single');
    FAD = typecast(rxdata(16:17),'uint16');
    elseif(modes == 6)
    VAmp = rxdata(6);
    VPW = typecast(rxdata(7:10),'single');
    AAmp = rxdata(11);
    APW = typecast(rxdata(12:15),'single');
    FAD = typecast(rxdata(16:17),'uint16');
    MAX_Sensor_Rate = rxdata(18);
    Reaction_Time = rxdata(19);
    Res_Factor = rxdata(20);
    Recovery_Time = rxdata(21);
    elseif(modes == 7)
    AAmp = rxdata(6);
    APW = typecast(rxdata(7:10),'single');
    ARP = typecast(rxdata(11:12),'uint16');
    MAX_Sensor_Rate = rxdata(13);
    Reaction_Time = rxdata(14);
    Res_Factor = rxdata(15);
    Recovery_Time = rxdata(16);
    AS = typecast(rxdata(17:20),'single');
    elseif(modes == 8)
    VAmp = rxdata(6);
    VPW = typecast(rxdata(7:10),'single');
    VRP = typecast(rxdata(11:12),'uint16');
    MAX_Sensor_Rate = rxdata(13);
    Reaction_Time = rxdata(14);
    Res_Factor = rxdata(15);
    Recovery_Time = rxdata(16);
    VS = typecast(rxdata(17:20),'single');
    elseif(modes == 9)
    AAmp = rxdata(6);
    APW = typecast(rxdata(7:10),'single');
    MAX_Sensor_Rate = rxdata(11);
    Reaction_Time = rxdata(12);
    Res_Factor = rxdata(13);
    Recovery_Time = rxdata(14);
    elseif(modes == 10)
    VAmp = rxdata(6);
    VPW = typecast(rxdata(7:10),'single');
    MAX_Sensor_Rate = rxdata(11);
    Reaction_Time = rxdata(12);
    Res_Factor = rxdata(13);
    Recovery_Time = rxdata(14);
    end
  state eegram
    entry:
    send_paramf();
  state ini
    entry:
    modes = 0;
    LRL = 60;
    URL = 120;
    AAmp = 70;
    VAmp = 70;
    APW = 1;
    VPW =1 ;
    ARP = 250;
    VRP = 320;
    FAD = 150;
    MAX_Sensor_Rate = 120;
    Reaction_Time = 30;
    Res_Factor = 8;
    Recovery_Time = 5;
    AS = 0;
    VS = 0;
  eegram -> (junction 61)
  (junction 18) -> eegram [order 2] : [rxdata(2)==34]
  (default) -> ini
  (junction 16) -> (junction 18) : [rxdata(1)==22]
  (junction 18) -> set1 [order 1] : [rxdata(2)==85]
  (junction 61) -> (junction 16) : [status==0]
  ini -> (junction 61)
  set1 -> (junction 61)
  data: rxdata input uint8 size=[21;1]; status input uint8 size=[1]; modes output uint8; LRL output uint8; AAmp output uint8; VAmp output uint8; APW output single size=[1;1]; VPW output single size=[1;1]; ARP output uint16 size=[1;1]; VRP output uint16 size=[1;1]; FAD output uint16 size=[1;1]; MAX_Sensor_Rate output uint8; Reaction_Time output uint8; Res_Factor output uint8; Recovery_Time output uint8; URL output uint8; AS output single size=[1;1]; VS output single size=[1;1]
